simulink model "FIR_FILTER"  (R2016a)
settings: Solver=VariableStepAuto  StartTime=0.0  StopTime=10.0  RelTol=1e-3
settings Model: Creator=HP  LastModifiedBy=HP

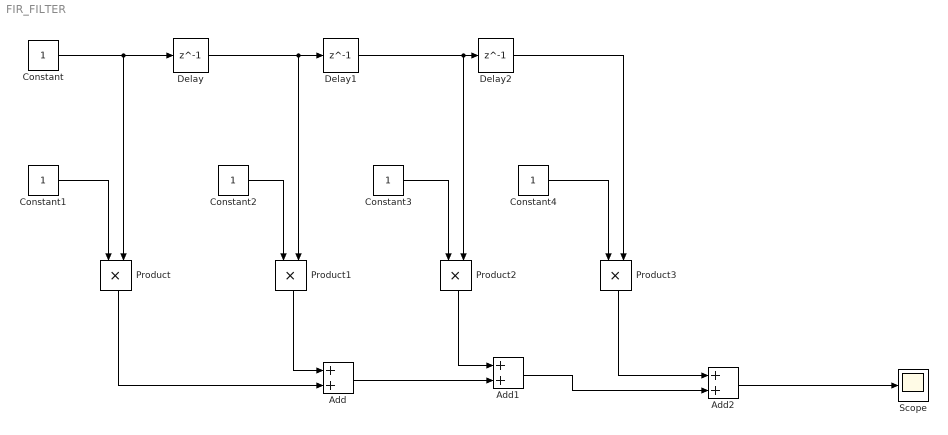
== system FIR_FILTER ==
  Add : Sum
  Add1 : Sum
  Add2 : Sum
  Constant : Constant  SampleTime=1
  Constant{1..4} (4 alike) : Constant
  Delay : Delay  DelayLength=1  InitialCondition=0
  Delay1 : Delay  DelayLength=1  InitialCondition=0
  Delay2 : Delay  DelayLength=1  InitialCondition=0
  Product{,1..3} (4 alike) : Product
  Scope : Scope
  wires:
  Constant/1 -> Delay/1, Product/2
  Delay/1 -> Product1/2, Delay1/1
  Delay1/1 -> Product2/2, Delay2/1
  Constant1/1 -> Product/1
  Constant2/1 -> Product1/1
  Constant3/1 -> Product2/1
  Constant4/1 -> Product3/1
  Delay2/1 -> Product3/2
  Product1/1 -> Add/1
  Product/1 -> Add/2
  Product2/1 -> Add1/1
  Add/1 -> Add1/2
  Product3/1 -> Add2/1
  Add1/1 -> Add2/2
  Add2/1 -> Scope/1
